simulink model "bonus"  (R2020a)
settings: Solver=ode45  StartTime=0.0  StopTime=10  RelTol=1e-8
settings Model: Creator=dot  LastModifiedBy=dot

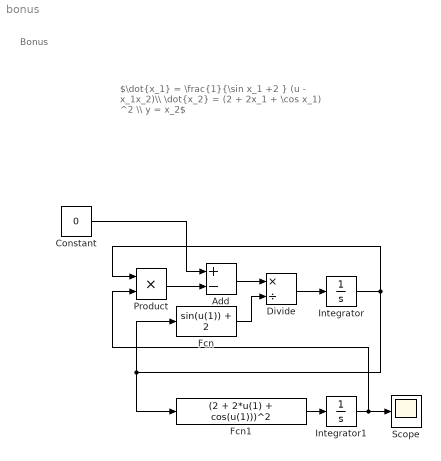
== system bonus ==
  note: Bonus
  note: $\dot{x_1} = \frac{1}{\sin x_1 +2 } (u - x_1x_2)\\ \dot{x_2} = (2 + 2x_1 + \cos x_1) ^2 \\ y = x_2$
  Add : Sum  Inputs=+-
  Constant : Constant  Value=0
  Divide : Product  Inputs=*/
  Fcn : Fcn  Expr=sin(u(1)) + 2
  Fcn1 : Fcn  Expr=(2 + 2*u(1) + cos(u(1)))^2
  Integrator : Integrator  InitialCondition=-1.18715
  Integrator1 : Integrator
  Product : Product
  Scope : Scope
  wires:
  Product/1 -> Add/2
  Add/1 -> Divide/1
  Divide/1 -> Integrator/1
  Integrator/1 -> Fcn1/1, Fcn/1, Product/1
  Constant/1 -> Add/1
  Fcn/1 -> Divide/2
  Integrator1/1 -> Scope/1, Product/2
  Fcn1/1 -> Integrator1/1
